simulink model "winter_simulink"  (R2022a)
settings: Solver=VariableStepAuto  StartTime=0.1  StopTime=30  FixedStep=sample_time/10  RelTol=1e-3
values from neighbouring files (symbols this model uses):
  B_eq = rotor.B + generator.B/gearbox.ratio^2    [parameters.m]
  I_eq = rotor.I + generator.I/gearbox.ratio^2    [parameters.m]
  lambda_opt = lambda_vector(lambda_pos)    [lookup_cp.m]    (also in mesh_cp.m; parameters.m = rated_values(4); reference_selection.m = 7.857)
  lambda_vector = linspace(lambda_range(1), lambda_range(2), lambda_item)    [mesh_cp.m]    (also in parameters.m)
  omega_rated = V0_rated*lambda_opt/rotor.R    [lookup_cp.m]    (also in mesh_cp.m; parameters.m = rated_values(2); reference_selection.m = 1.008234212)
  pitch_vector = linspace(pitch_range(1), pitch_range(2), pitch_item)    [mesh_cp.m]    (also in parameters.m)
  rho = 1.225    [parameters.m]    (also in reference_selection.m)
  sample_time = wind_speed(2,1) - wind_speed(1, 1)    [parameters.m]
  V0_rated = (rotor.P_rated/(0.5*rho*cP_max*rotor.A))^(1/3)    [lookup_cp.m]    (also in mesh_cp.m; parameters.m = rated_values(1); reference_selection.m = 11.44)
  wind_speed = WS(i)    [main.m]    (also in parameters.m = load('usim.dat'); rotor_test.m = 25)
undefined symbols (not defined in the file or in its folder): blade, gearbox, generator, lookup_cP, omega_r, rotor
settings Model: Creator=Niccolò  LastModifiedBy=Niccolò

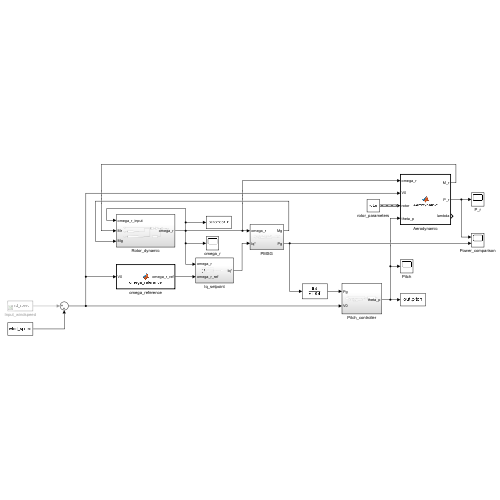
[thumbnail: Simulink's stored preview of the top-level diagram]
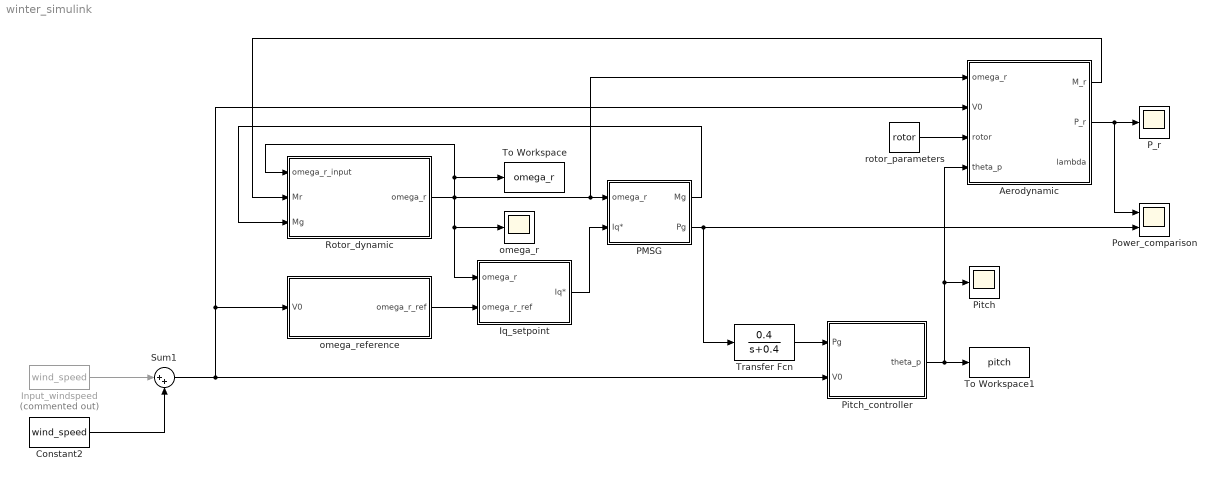
== system winter_simulink ==
  Aerodynamic : MATLAB Function  TreatAsAtomicUnit=on
  Constant2 : Constant  Value=wind_speed
  Input_windspeed : FromWorkspace  Commented=on  VariableName=wind_speed  SampleTime=sample_time
  Iq_setpoint : Subsystem
  PMSG : Subsystem
  P_r : Scope
  Pitch : Scope
  Pitch_controller : Subsystem
  Power_comparison : Scope  NumInputPorts=2
  Rotor_dynamic : Subsystem
  Sum1 : Sum  Inputs=|++
  To Workspace : ToWorkspace  VariableName=omega_r  SaveFormat=Timeseries  SampleTime=-1
  To Workspace1 : ToWorkspace  VariableName=pitch  SaveFormat=Timeseries  SampleTime=-1
  Transfer Fcn : TransferFcn  Numerator=[0.4]  Denominator=[1 0.4]
  omega_r : Scope
  omega_reference : MATLAB Function  TreatAsAtomicUnit=on
  rotor_parameters : Constant  Value=rotor  OutDataTypeStr=Bus: rotor_bus
  wires:
  PMSG/2(Pg) -> Transfer Fcn/1, Power_comparison/2
  Aerodynamic/2(P_r) -> P_r/1, Power_comparison/1
  Input_windspeed/1 -> Sum1/1
  rotor_parameters/1 -> Aerodynamic/3(rotor)
  Pitch_controller/1(theta_p) -> To Workspace1/1, Aerodynamic/4(theta_p), Pitch/1
  Constant2/1 -> Sum1/2
  omega_reference/1(omega_r_ref) -> Iq_setpoint/2(omega_r_ref)
  Aerodynamic/1(M_r) -> Rotor_dynamic/2(Mr)
  PMSG/1(Mg) -> Rotor_dynamic/3(Mg)
  Iq_setpoint/1(Iq*) -> PMSG/2(Iq*)
  Rotor_dynamic/1(omega_r) -> Iq_setpoint/1(omega_r), omega_r/1, Aerodynamic/1(omega_r), PMSG/1(omega_r), Rotor_dynamic/1(omega_r_input), To Workspace/1
  Transfer Fcn/1 -> Pitch_controller/1(Pg)
  Sum1/1 -> Aerodynamic/2(V0), omega_reference/1(V0), Pitch_controller/2(V0)

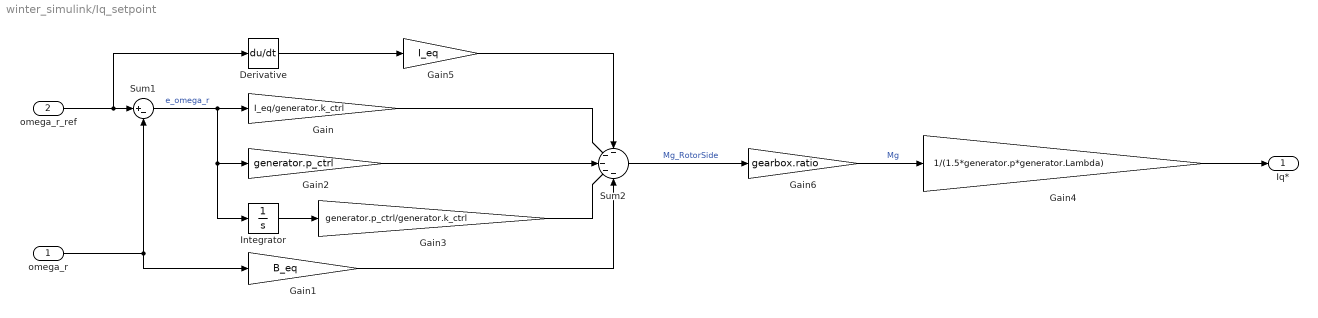
== system winter_simulink/Iq_setpoint ==
  omega_r : Inport
  omega_r_ref : Inport  Port=2
  Derivative : Derivative
  Gain : Gain  Gain=I_eq/generator.k_ctrl
  Gain1 : Gain  Gain=B_eq
  Gain2 : Gain  Gain=generator.p_ctrl
  Gain3 : Gain  Gain=generator.p_ctrl/generator.k_ctrl
  Gain4 : Gain  Gain=1/(1.5*generator.p*generator.Lambda)
  Gain5 : Gain  Gain=I_eq
  Gain6 : Gain  Gain=gearbox.ratio
  Integrator : Integrator
  Sum1 : Sum  Inputs=|+-
  Sum2 : Sum  Inputs=-----
  Iq* : Outport
  wires:
  Gain/1 -> Sum2/2
  Sum1/1 -> Integrator/1, Gain2/1, Gain/1  "e_omega_r"
  Gain1/1 -> Sum2/5
  Gain4/1 -> Iq*/1
  omega_r_ref/1 -> Derivative/1, Sum1/1
  omega_r/1 -> Gain1/1, Sum1/2
  Integrator/1 -> Gain3/1
  Gain3/1 -> Sum2/4
  Gain2/1 -> Sum2/3
  Sum2/1 -> Gain6/1  "Mg_RotorSide"
  Gain5/1 -> Sum2/1
  Gain6/1 -> Gain4/1  "Mg"
  Derivative/1 -> Gain5/1

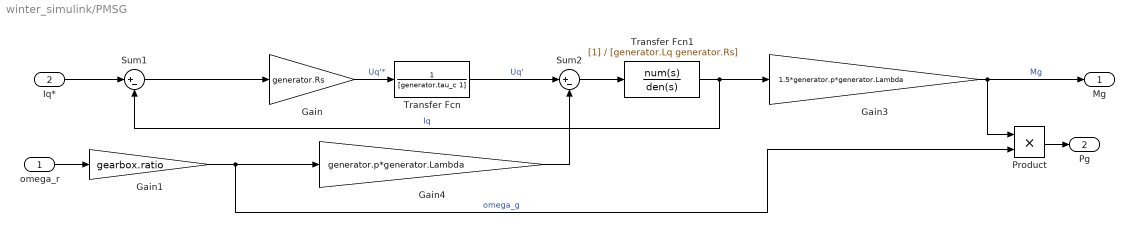
== system winter_simulink/PMSG ==
  omega_r : Inport
  Iq* : Inport  Port=2
  Gain : Gain  Gain=generator.Rs
  Gain1 : Gain  Gain=gearbox.ratio
  Gain3 : Gain  Gain=1.5*generator.p*generator.Lambda
  Gain4 : Gain  Gain=generator.p*generator.Lambda
  Product : Product
  Sum1 : Sum  Inputs=|+-
  Sum2 : Sum  Inputs=|+-
  Transfer Fcn : TransferFcn  Denominator=[generator.tau_c 1]
  Transfer Fcn1 : TransferFcn  Denominator=[generator.Lq generator.Rs]
  Mg : Outport
  Pg : Outport  Port=2
  wires:
  Sum2/1 -> Transfer Fcn1/1
  omega_r/1 -> Gain1/1
  Transfer Fcn1/1 -> Gain3/1, Sum1/2  "Iq"
  Sum1/1 -> Gain/1
  Transfer Fcn/1 -> Sum2/1  "Uq'"
  Gain/1 -> Transfer Fcn/1  "Uq'*"
  Gain4/1 -> Sum2/2
  Gain3/1 -> Product/1, Mg/1  "Mg"
  Iq*/1 -> Sum1/1
  Gain1/1 -> Product/2, Gain4/1  "omega_g"
  Product/1 -> Pg/1

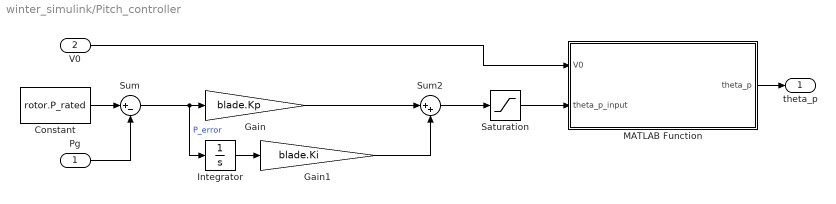
== system winter_simulink/Pitch_controller ==
  Pg : Inport
  V0 : Inport  Port=2
  Constant : Constant  Value=rotor.P_rated
  Gain : Gain  Gain=blade.Kp
  Gain1 : Gain  Gain=blade.Ki
  Integrator : Integrator
  MATLAB Function : MATLAB Function  TreatAsAtomicUnit=on
  Saturation : Saturate  UpperLimit=pi/2 - 0.1  LowerLimit=0
  Sum : Sum  Inputs=|+-
  Sum2 : Sum  Inputs=|++
  theta_p : Outport
  wires:
  Pg/1 -> Sum/2
  Sum/1 -> Integrator/1, Gain/1  "P_error"
  Constant/1 -> Sum/1
  Gain/1 -> Sum2/1
  Gain1/1 -> Sum2/2
  Integrator/1 -> Gain1/1
  V0/1 -> MATLAB Function/1(V0)
  MATLAB Function/1(theta_p) -> theta_p/1
  Sum2/1 -> Saturation/1
  Saturation/1 -> MATLAB Function/2(theta_p_input)

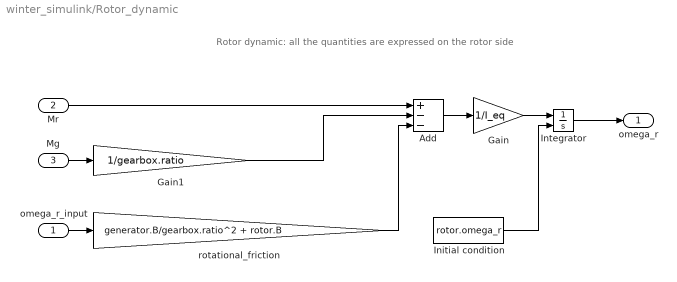
== system winter_simulink/Rotor_dynamic ==
  note: Rotor dynamic: all the quantities are expressed on the rotor side
  omega_r_input : Inport
  Mr : Inport  Port=2
  Mg : Inport  Port=3
  Add : Sum  Inputs=+--
  Gain : Gain  Gain=1/I_eq
  Gain1 : Gain  Gain=1/gearbox.ratio
  Initial condition : Constant  Value=rotor.omega_r
  Integrator : Integrator  InitialConditionSource=external  InitialCondition=omega_r
  rotational_friction : Gain  Gain=generator.B/gearbox.ratio^2 + rotor.B
  omega_r : Outport
  wires:
  Add/1 -> Gain/1
  Gain/1 -> Integrator/1
  Mr/1 -> Add/1
  Initial condition/1 -> Integrator/2
  omega_r_input/1 -> rotational_friction/1
  rotational_friction/1 -> Add/3
  Mg/1 -> Gain1/1
  Gain1/1 -> Add/2
  Integrator/1 -> omega_r/1

== matlab function winter_simulink/Pitch_controller/MATLAB Function ==
  data: theta_p output; V0 input; theta_p_input input; V0_rated parameter
function theta_p = theta_choice(V0, theta_p_input, V0_rated)

if V0 < V0_rated
  theta_p = 0.0;
else 
  theta_p = theta_p_input;
end

== matlab function winter_simulink/Aerodynamic ==
  data: omega_r input; V0 input; M_r output; P_r output; rho parameter; rotor input; theta_p input; lambda_vector parameter; pitch_vector parameter; lookup_cP parameter; lambda output
function [M_r, P_r, lambda] = Aerodynamic(omega_r, V0, rho, rotor, theta_p, ...
  lambda_vector, pitch_vector, lookup_cP) 

R = rotor.R;                  % rotor radius [m]

% retrive the cP from the look-up table
lambda = omega_r*R/V0;                                                
cP = interp2(lambda_vector, pitch_vector, lookup_cP, lambda, theta_p);

P_r = 0.5*rho*V0^3*pi*R^2*cP; % rotor power [W]
M_r = P_r/omega_r;            % rotor torque [Nm]

== matlab function winter_simulink/omega_reference ==
  data: V0 input; omega_r_ref output; lambda_opt parameter; rotor parameter; omega_rated parameter; V0_rated parameter
function omega_r_ref = omega_reference(V0, lambda_opt, rotor, ...
  omega_rated, V0_rated)
% This block provides the gnereator reference speed based on the expected
% rotor reference speed and the gearbox ratio

% rotor refernce speed
if V0 < V0_rated    % below rated -> MPPT
  omega_r_ref = lambda_opt*V0/rotor.R;
else                % above rated -> power limitation
  omega_r_ref = omega_rated;
end
